simulink model "q"  (R2020a)
settings: Solver=FixedStepAuto  StartTime=0.0  StopTime=10.0  FixedStep=1e-6  RelTol=1e-3  EnableMultiTasking=on
undefined symbols (not defined in the file or in its folder): A
libraries: powerlib x9, powerlib_meascontrol x1
settings Model: Creator=SINA  LastModifiedBy=ABO-CHIFA
settings DataIOCC: ReturnWorkspaceOutputs=off
settings OptimizationCC: LifeSpan=inf
settings DebuggingCC: SFUnexpectedBacktrackingDiag=warning  SFNoUnconditionalDefaultTransitionDiag=warning  ArithmeticOperatorsInVariantConditions=warning
settings SFSimCC: SimUseLocalCustomCode=off  CustomCodeUndefinedFunction=UseInterfaceOnly
settings RTWCC: RTWUseLocalCustomCode=off
settings CodeAppCC: StateflowObjectComments=on
settings GRTTargetCC: TargetLangStandard=C89/C90 (ANSI)
settings ConfigComp: CovMetricSettings=dw  CovHtmlReporting=on  CovSaveCumulativeToWorkspaceVar=on  CovSaveSingleToWorkspaceVar=on  CovExternalEMLEnable=off
settings SimscapeCC: SimscapeNormalizeSystem=off

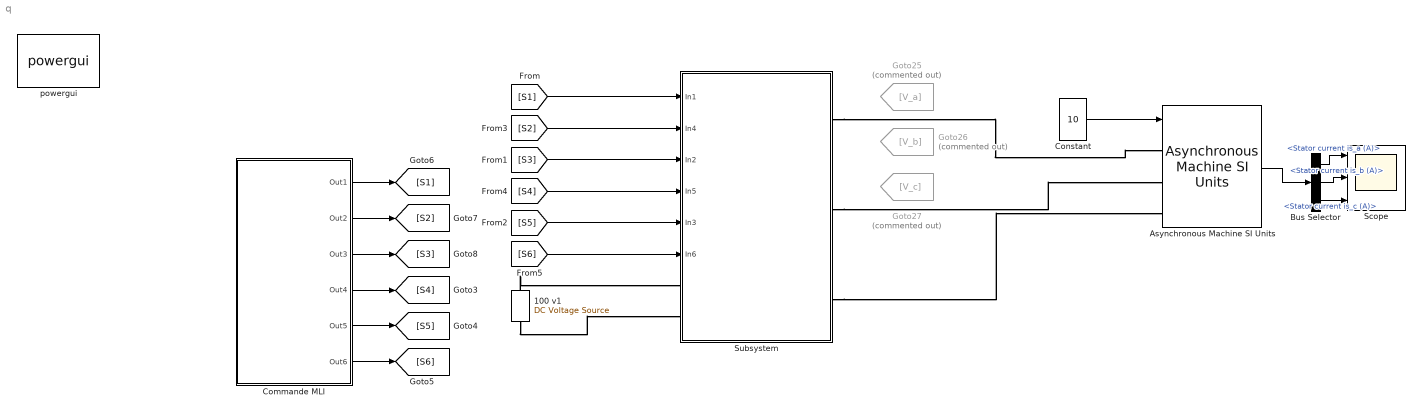
== system q ==
  100 v1 : powerlib/Electrical Sources/DC Voltage Source  Amplitude=220  Measurements=Voltage
  Asynchronous Machine SI Units : powerlib/Machines/Asynchronous Machine SI Units  RotorType=Squirrel-cage  PresetModel="15:  5.4 HP (4KW)   400 V  50Hz 1430 RPM"  MechanicalLoad=Torque Tm  ShowDetailedParameters=on  ReferenceFrame=Rotor  Units=SI  MeasurementBus=off  NominalParameters=[4000 400 50]  Stator=[1.405 0.005839]  Rotor=[1.395 0.005839]  Cage1=[0.4155 0.002066]  Cage2=[0.4168 0.0003495]  Lm=0.1722  Mechanical=[0.0131 0.002985 2]  PolePairs=2  InitialConditions=[1 0 0 0 0 0 0 0]  SimulateSaturation=off  Saturation=[14.03593122, 27.81365428, 53.79336849, 72.68890987, 97.98006896, 148.6815601, 215.7428561, 302.9841135, 428.7778367 ; 230, 322, 414, 460, 506, 552, 598, 644, 690]  LoadFlowParameters=1492000  TsPowergui=0  TsBlock=-1  IterativeModel=Trapezoidal non iterative  IterativeDiscreteModel=Trapezoidal non iterative  Pmec=1.492e+006
  Bus Selector : BusSelector  OutputSignals=Stator measurements.Stator current is_a (A),Stator measurements.Stator current is_b (A),Stator measurements.Stator current is_c (A)
  "Commande MLI " : Subsystem
  Constant : Constant  Value=10
  Goto25 : Goto  Commented=on  GotoTag=V_a
  Goto26 : Goto  Commented=on  GotoTag=V_b
  Goto27 : Goto  Commented=on  GotoTag=V_c
  Scope : Scope  NumInputPorts=3
  Subsystem : Subsystem
  powergui : powerlib/powergui  Priority=1  SimulationMode=Discrete  SampleTime=1e-6  frequency=60  Iterations=50  frequencyindice=0  Pbase=100e6  ErrMax=1e-4  UnitsV=kV  UnitsW=MW  buscounter=0  FunctionMessages=off  echomessages=off  EnableUseOfTLC=off  CurrentSourceSwitches=off  DisableSnubberDevices=off  DisableRonSwitches=off  DisableVfSwitches=off  DisplayEquations=off  AutomaticDiscreteSolvers=off  SolverType=Tustin/Backward Euler (TBE)  Interpol=off  ExternalGateDelay=off  methode=off  Ts=10  x0status=blocks  SPID=off  SwTol=0  HookPort=off  NonlinearTolerance=1e-4  nMaxIteration=100  ContinueOnMaxIteration=off  RestoreLinks=warning  ResistiveCurrentMeasurement=off  Frange=[0:2:500]  Ylog=off  Xlog=on  ShowGrid=off  save=off  variable=ZData  structure=0  ZoomFFT=off  StartTime=0.0  cycles=1  DisplayStyle=1  fundamental=60  FreqAxis=off  MaxFrequency=1000  frequencyindicesteady=1  RmsSteady=1  display=off
  wires:
  "Commande MLI "/4(Out4) -> [S4]
  "Commande MLI "/5(Out5) -> [S5]
  "Commande MLI "/6(Out6) -> [S6]
  "Commande MLI "/2(Out2) -> [S2]
  "Commande MLI "/1(Out1) -> [S1]
  "Commande MLI "/3(Out3) -> [S3]
  [S1] -> Subsystem/1(In1)
  [S3] -> Subsystem/3(In2)
  [S5] -> Subsystem/5(In3)
  [S2] -> Subsystem/2(In4)
  [S4] -> Subsystem/4(In5)
  [S6] -> Subsystem/6(In6)
  Constant/1 -> Asynchronous Machine SI Units/1
  Asynchronous Machine SI Units/1 -> Bus Selector/1
  Bus Selector/1 -> Scope/1  "<Stator current is_a (A)>"
  Bus Selector/2 -> Scope/2  "<Stator current is_b (A)>"
  Bus Selector/3 -> Scope/3  "<Stator current is_c (A)>"
  connections:
  Subsystem/RConn3 -- Asynchronous Machine SI Units/LConn3
  Subsystem/RConn2 -- Asynchronous Machine SI Units/LConn2
  Subsystem/RConn1 -- Asynchronous Machine SI Units/LConn1
  100 v1/RConn1 -- Subsystem/LConn1
  100 v1/LConn1 -- Subsystem/LConn2

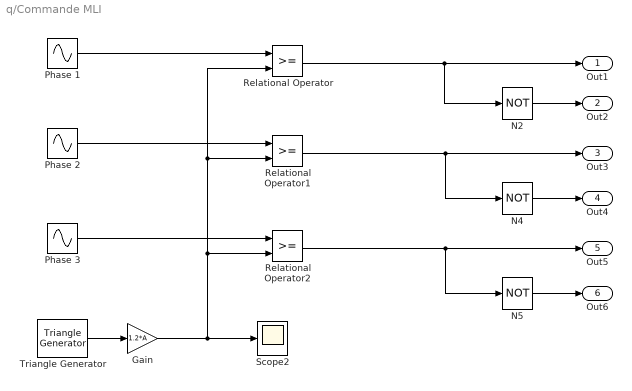
== system q/Commande MLI  ==
  Gain : Gain  Gain=1.2*A
  N2 : Logic  Operator=NOT  AllPortsSameDT=off  OutDataTypeStr=boolean
  N4 : Logic  Operator=NOT  AllPortsSameDT=off  OutDataTypeStr=boolean
  N5 : Logic  Operator=NOT  AllPortsSameDT=off  OutDataTypeStr=boolean
  "Phase 1 " : Sin  Amplitude=220  Frequency=2*pi*50  SampleTime=0
  Phase 2 : Sin  Amplitude=220  Frequency=2*pi*50  Phase=-2*pi/3  SampleTime=0
  Phase 3 : Sin  Amplitude=220  Frequency=2*pi*50  Phase=2*pi/3  SampleTime=0
  Relational Operator : RelationalOperator  OutDataTypeStr=boolean  RndMeth=Nearest
  Relational Operator1 : RelationalOperator  OutDataTypeStr=boolean  RndMeth=Nearest
  Relational Operator2 : RelationalOperator  OutDataTypeStr=boolean  RndMeth=Nearest
  Scope2 : Scope
  Triangle Generator : powerlib_meascontrol/Pulse & Signal Generators/Triangle Generator  Freq=1e3  Phase=90  Ts=0
  Out1 : Outport
  Out2 : Outport  Port=2
  Out3 : Outport  Port=3
  Out4 : Outport  Port=4
  Out5 : Outport  Port=5
  Out6 : Outport  Port=6
  wires:
  Phase 3/1 -> Relational Operator2/1
  N4/1 -> Out4/1
  N5/1 -> Out6/1
  N2/1 -> Out2/1
  Relational Operator/1 -> N2/1, Out1/1
  Relational Operator1/1 -> Out3/1, N4/1
  Relational Operator2/1 -> Out5/1, N5/1
  Phase 2/1 -> Relational Operator1/1
  "Phase 1 "/1 -> Relational Operator/1
  Triangle Generator/1 -> Gain/1
  Gain/1 -> Relational Operator2/2, Relational Operator1/2, Relational Operator/2, Scope2/1

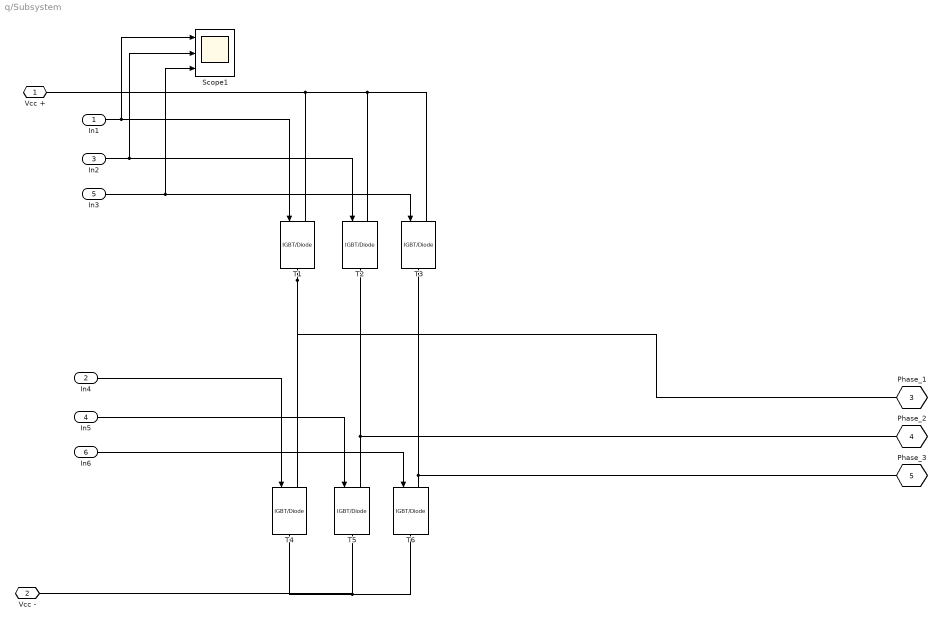
== system q/Subsystem ==
  In1 : Inport
  In4 : Inport  Port=2
  In2 : Inport  Port=3
  In5 : Inport  Port=4
  In3 : Inport  Port=5
  In6 : Inport  Port=6
  Scope1 : Scope  NumInputPorts=3
  T{1..6} (6 alike) : powerlib/Power Electronics/IGBT//Diode  Ron=1e-3  Rs=1e5  Cs=inf  Measurements=off
  Vcc + : PMIOPort  Side=Left
  Vcc - : PMIOPort  Port=2  Side=Left
  Phase_1 : PMIOPort  Tag=PMCPort  Port=3  Side=Right
  Phase_2 : PMIOPort  Tag=PMCPort  Port=4  Side=Right
  Phase_3 : PMIOPort  Tag=PMCPort  Port=5  Side=Right
  wires:
  In1/1 -> Scope1/1, T1/1
  In2/1 -> Scope1/2, T2/1
  In3/1 -> Scope1/3, T3/1
  In4/1 -> T4/1
  In5/1 -> T5/1
  In6/1 -> T6/1
  connections:
  T2/LConn1 -- T3/LConn1 -- Vcc +/RConn1 -- T1/LConn1
  T5/RConn1 -- T4/RConn1 -- Vcc -/RConn1 -- T6/RConn1
  T1/RConn1 -- Phase_1/RConn1 -- T4/LConn1
  T5/LConn1 -- T2/RConn1 -- Phase_2/RConn1
  T6/LConn1 -- T3/RConn1 -- Phase_3/RConn1
